simulink model "Waterflow"  (R2016a)
settings: Solver=VariableStepAuto  StartTime=0.0  StopTime=10.0  RelTol=1e-3
settings Model: Creator=Pection  LastModifiedBy=Pection

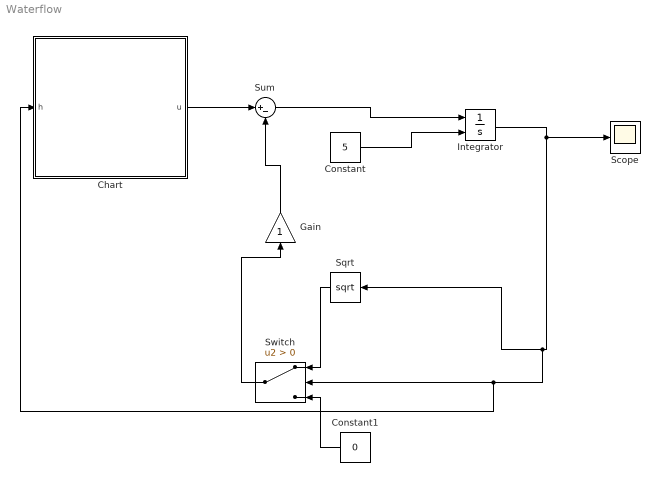
== system Waterflow ==
  Chart : Stateflow chart  TreatAsAtomicUnit=on
  Constant : Constant  Value=5
  Constant1 : Constant  Value=0
  Gain : Gain
  Integrator : Integrator  InitialConditionSource=external
  Scope : Scope
  Sqrt : Sqrt  SaturateOnIntegerOverflow=on
  Sum : Sum  Inputs=|+-
  Switch : Switch  Criteria=u2 > Threshold
  wires:
  Integrator/1 -> Scope/1, Chart/1(h), Switch/2, Sqrt/1
  Sum/1 -> Integrator/1
  Gain/1 -> Sum/2
  Constant/1 -> Integrator/2
  Sqrt/1 -> Switch/1
  Constant1/1 -> Switch/3
  Switch/1 -> Gain/1
  Chart/1(u) -> Sum/1

== stateflow chart Waterflow/Chart ==
  state Below
    during:
    u=10;
  state Above
    during:
    u=0;
  state Medium
  Medium -> Below [order 2] : [h<=2.5]
  (default) -> Above
  Below -> Medium : [h>2.5]
  Above -> Medium : [h<=7.5]
  Medium -> Above [order 1] : [h>7.5]
  data: h input; u output
